simulink model "OpenLoop"  (Simulink 10.2)
settings: Solver=ode4  StartTime=0.0  StopTime=TMax  FixedStep=DT  MaxStep=DT  RelTol=1e-3  EnableMultiTasking=on
undefined symbols (not defined in the file or in its folder): OutList, sigbuilder_block, strmatch
settings Model: LogicAnalyzerSignalOrdering=622969c7-4a95-484c-aa48-d70039800655,567f855e-93bb-40e6-82fe-fffaa7f8c6d2,f9a8c3cb-64e9-4f89-868b-cd3825c112bf,cfa72df4-fa35-4a41-bc9f-f1a82cc1069a,cd711ec8-28aa-4c52-819f-5cc7fce55bd0  Creator=bjonkman  LastModifiedBy=oster
settings DataIOCC: LimitDataPoints=on  SaveOutput=off  SaveTime=off  SignalLoggingName=sigsOut
settings OptimizationCC: ExpressionDepthLimit=2147483647
settings DebuggingCC: SaveWithParameterizedLinksMsg=none  SignalResolutionControl=TryResolveAllWithWarning  MultiTaskDSMMsg=warning  MultiTaskCondExecSysMsg=none  StateNameClashWarn=warning
settings HardwareCC: TargetUnknown=on

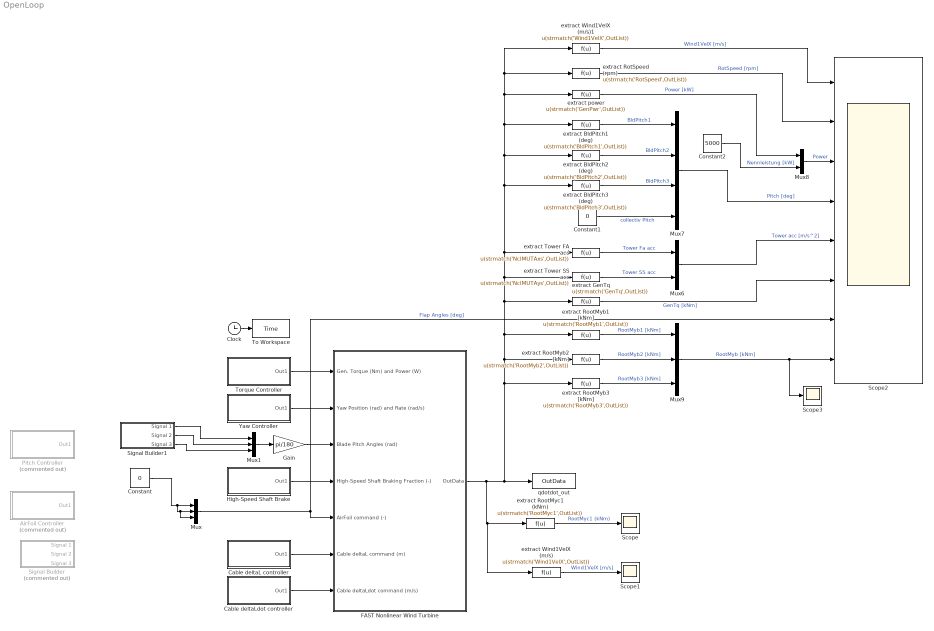
== system OpenLoop ==
  AirFoil Controller : Subsystem  Commented=on
  Cable deltaL controller : Subsystem
  Cable deltaLdot controller : Subsystem
  Clock : Clock
  Constant : Constant  Value=0
  Constant1 : Constant  Value=0
  Constant2 : Constant  Value=5000
  FAST Nonlinear Wind Turbine : Subsystem  mask(FAST Nonlinear Wind Turbine){}
      mask help: This block contains the FAST S-Function.
      mask init:
      | clear FAST_SFunc
  Gain : Gain  Gain=pi/180
  High-Speed Shaft Brake : Subsystem
  Mux : Mux  Inputs=3
  Mux1 : Mux  Inputs=3
  Mux6 : Mux  Inputs=2
  Mux7 : Mux
  Mux8 : Mux  Inputs=2
  Mux9 : Mux  Inputs=3
  Pitch Controller : Subsystem  Commented=on
  Scope : Scope
  Scope1 : Scope
  Scope2 : Scope  NumInputPorts=8
  Scope3 : Scope
  Signal Builder : Subsystem  Tag=STV Subsys  Commented=on  LoadFcn=sigbuilder_block('load');  StartFcn=sigbuilder_block('start');  StopFcn=sigbuilder_block('stop');  ClipboardFcn=sigbuilder_block('clipboard');  mask(Sigbuilder block){tuvar=[0:10]}
      mask help: Simulink:masks:SigbuilderBlock_MD
      mask init:
      | if ~strcmp(get_param(bdroot(gcbh),'SimulationStatus'),'stopped') tuvar = sigbuilder_block('maskInit'); end
      settings: CopyFcn=sigbuilder_block('copy');  DeleteFcn=sigbuilder_block('delete');  ModelCloseFcn=sigbuilder_block('modelClose');  PreSaveFcn=sigbuilder_block('preSave');  PauseFcn=sigbuilder_block('pause');  ContinueFcn=sigbuilder_block('continue');  NameChangeFcn=sigbuilder_block('namechange');  OpenFcn=sigbuilder_block('open',[1778.25 246.75 675 420.75 ]);  CloseFcn=sigbuilder_block('close');
      mask Display: plot(0, 0, 100, 100,[2, 2, 32, 32, 2], [68, 8, 8, 68, 68],[32, 2], [38, 38], [32, 19, 2],[53, 60, 44], [32, 17, 17, 2],[16, 16, 31, 31]);txt = getActiveGroup(gcbh);text(2, 100, txt,'verticalAlignment', 'top');
  Signal Builder1 : Subsystem  Tag=STV Subsys  LoadFcn=sigbuilder_block('load');  StartFcn=sigbuilder_block('start');  StopFcn=sigbuilder_block('stop');  ClipboardFcn=sigbuilder_block('clipboard');  mask(Sigbuilder block){tuvar=[0:10]}
      mask help: Simulink:masks:SigbuilderBlock_MD
      mask init:
      | if ~strcmp(get_param(bdroot(gcbh),'SimulationStatus'),'stopped') tuvar = sigbuilder_block('maskInit'); end
      settings: CopyFcn=sigbuilder_block('copy');  DeleteFcn=sigbuilder_block('delete');  ModelCloseFcn=sigbuilder_block('modelClose');  PreSaveFcn=sigbuilder_block('preSave');  PauseFcn=sigbuilder_block('pause');  ContinueFcn=sigbuilder_block('continue');  NameChangeFcn=sigbuilder_block('namechange');  OpenFcn=sigbuilder_block('open',[1778.25 246.75 675 420.75 ]);  CloseFcn=sigbuilder_block('close');
      mask Display: plot(0, 0, 100, 100,[2, 2, 32, 32, 2], [68, 8, 8, 68, 68],[32, 2], [38, 38], [32, 19, 2],[53, 60, 44], [32, 17, 17, 2],[16, 16, 31, 31]);txt = getActiveGroup(gcbh);text(2, 100, txt,'verticalAlignment', 'top');
  To Workspace : ToWorkspace  VariableName=Time  SampleTime=-1
  Torque Controller : Subsystem
  Yaw Controller : Subsystem
  extract BldPitch1 (deg) : Fcn  Expr=u(strmatch('BldPitch1',OutList))
  extract BldPitch2 (deg) : Fcn  Expr=u(strmatch('BldPitch2',OutList))
  extract BldPitch3 (deg) : Fcn  Expr=u(strmatch('BldPitch3',OutList))
  extract GenTq : Fcn  Expr=u(strmatch('GenTq',OutList))
  extract RootMyb1 [kNm] : Fcn  Expr=u(strmatch('RootMyb1',OutList))
  extract RootMyb2 [kNm] : Fcn  Expr=u(strmatch('RootMyb2',OutList))
  extract RootMyb3 [kNm] : Fcn  Expr=u(strmatch('RootMyb3',OutList))
  extract RootMyc1 (kNm) : Fcn  Expr=u(strmatch('RootMyc1',OutList))
  extract RotSpeed (rpm) : Fcn  Expr=u(strmatch('RotSpeed',OutList))
  extract Tower FA acc : Fcn  Expr=u(strmatch('NcIMUTAxs',OutList))
  extract Tower SS acc : Fcn  Expr=u(strmatch('NcIMUTAys',OutList))
  extract Wind1VelX (m/s) : Fcn  Expr=u(strmatch('Wind1VelX',OutList))
  extract Wind1VelX (m/s)1 : Fcn  Expr=u(strmatch('Wind1VelX',OutList))
  extract power : Fcn  Expr=u(strmatch('GenPwr',OutList))
  qdotdot_out : ToWorkspace  VariableName=OutData  SampleTime=-1
  wires:
  Clock/1 -> To Workspace/1
  Torque Controller/1(Out1) -> FAST Nonlinear Wind Turbine/1(Gen. Torque (Nm) and Power (W))
  Yaw Controller/1(Out1) -> FAST Nonlinear Wind Turbine/2(Yaw Position (rad) and Rate (rad/s))
  Mux1/1 -> Gain/1
  High-Speed Shaft Brake/1(Out1) -> FAST Nonlinear Wind Turbine/4(High-Speed Shaft Braking Fraction (-))
  Cable deltaL controller/1(Out1) -> FAST Nonlinear Wind Turbine/6(Cable deltaL command (m))
  Cable deltaLdot controller/1(Out1) -> FAST Nonlinear Wind Turbine/7(Cable deltaLdot command (m/s))
  extract RootMyc1 (kNm)/1 -> Scope/1  "RootMyc1 (kNm)"
  extract Wind1VelX (m/s)/1 -> Scope1/1  "Wind1VelX [m/s]"
  extract Tower FA acc/1 -> Mux6/1  "Tower Fa acc"
  extract BldPitch2 (deg)/1 -> Mux7/2  "BldPitch2"
  extract Wind1VelX (m/s)1/1 -> Scope2/1  "Wind1VelX [m/s]"
  extract GenTq/1 -> Scope2/6  "GenTq [kNm]"
  extract RootMyb1 [kNm]/1 -> Mux9/1  "RootMyb1 [kNm]"
  Mux6/1 -> Scope2/5  "Tower acc [m/s^2]"
  extract RootMyb3 [kNm]/1 -> Mux9/3  "RootMyb3 [kNm]"
  extract BldPitch1 (deg)/1 -> Mux7/1  "BldPitch1"
  extract RotSpeed (rpm)/1 -> Scope2/2  "RotSpeed [rpm]"
  extract BldPitch3 (deg)/1 -> Mux7/3  "BldPitch3"
  extract Tower SS acc/1 -> Mux6/2  "Tower SS acc"
  FAST Nonlinear Wind Turbine/1(OutData) -> extract Wind1VelX (m/s)/1, extract RootMyc1 (kNm)/1, extract RootMyb3 [kNm]/1, extract RootMyb1 [kNm]/1, extract GenTq/1, extract Tower SS acc/1, extract Tower FA acc/1, extract RotSpeed (rpm)/1, extract Wind1VelX (m/s)1/1, extract power/1, extract BldPitch1 (deg)/1, extract BldPitch2 (deg)/1, extract BldPitch3 (deg)/1, extract RootMyb2 [kNm]/1, qdotdot_out/1
  Constant1/1 -> Mux7/4  "collectiv Pitch"
  Constant2/1 -> Mux8/2  "Nennleistung [kW]"
  Mux/1 -> FAST Nonlinear Wind Turbine/5(AirFoil command (-)), Scope2/7  "Flap Angles [deg]"
  extract RootMyb2 [kNm]/1 -> Mux9/2  "RootMyb2 [kNm]"
  Mux9/1 -> Scope3/1, Scope2/8  "RootMyb [kNm]"
  extract power/1 -> Mux8/1  "Power [kW]"
  Mux8/1 -> Scope2/3  "Power"
  Mux7/1 -> Scope2/4  "Pitch [deg]"
  Signal Builder1/3(Signal 3) -> Mux1/3
  Signal Builder1/2(Signal 2) -> Mux1/2
  Signal Builder1/1(Signal 1) -> Mux1/1
  Constant/1 -> Mux/3, Mux/2, Mux/1
  Gain/1 -> FAST Nonlinear Wind Turbine/3(Blade Pitch Angles (rad))

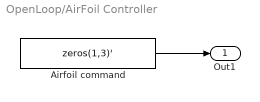
== system OpenLoop/AirFoil Controller ==
  Airfoil command : Constant  Value=zeros(1,3)'
  Out1 : Outport
  wires:
  Airfoil command/1 -> Out1/1

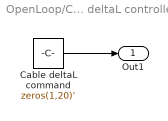
== system OpenLoop/Cable deltaL controller ==
  Cable deltaL command : Constant  Value=zeros(1,20)'
  Out1 : Outport
  wires:
  Cable deltaL command/1 -> Out1/1

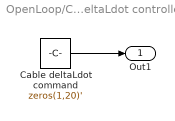
== system OpenLoop/Cable deltaLdot controller ==
  Cable deltaLdot command : Constant  Value=zeros(1,20)'
  Out1 : Outport
  wires:
  Cable deltaLdot command/1 -> Out1/1

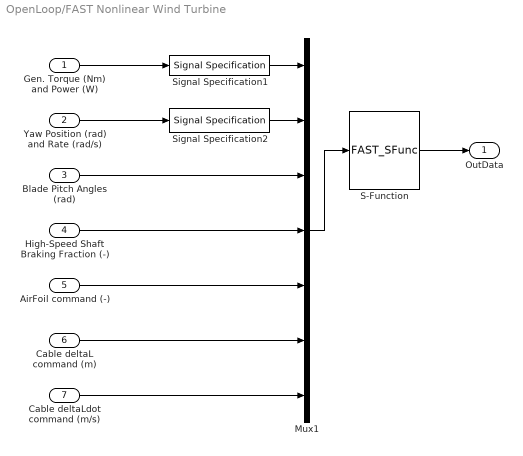
== system OpenLoop/FAST Nonlinear Wind Turbine ==
  Gen. Torque (Nm) and Power (W) : Inport
  Yaw Position (rad) and Rate (rad/s) : Inport  Port=2
  Blade Pitch Angles (rad) : Inport  Port=3
  High-Speed Shaft Braking Fraction (-) : Inport  Port=4
  AirFoil command (-) : Inport  Port=5
  Cable deltaL command (m) : Inport  Port=6
  Cable deltaLdot command (m/s) : Inport  Port=7
  Mux1 : Mux  Inputs=7
  S-Function : S-Function  FunctionName=FAST_SFunc  Parameters=FAST_InputFileName, TMax, 0  SFunctionDeploymentMode=off  EnableBusSupport=off
  Signal Specification1 : SignalSpecification  OutDataTypeStr=double  Dimensions=2
  Signal Specification2 : SignalSpecification  OutDataTypeStr=double  Dimensions=2
  OutData : Outport
  wires:
  Gen. Torque (Nm) and Power (W)/1 -> Signal Specification1/1
  S-Function/1 -> OutData/1
  Mux1/1 -> S-Function/1
  Blade Pitch Angles (rad)/1 -> Mux1/3
  Yaw Position (rad) and Rate (rad/s)/1 -> Signal Specification2/1
  Signal Specification1/1 -> Mux1/1
  Signal Specification2/1 -> Mux1/2
  High-Speed Shaft Braking Fraction (-)/1 -> Mux1/4
  AirFoil command (-)/1 -> Mux1/5
  Cable deltaL command (m)/1 -> Mux1/6
  Cable deltaLdot command (m/s)/1 -> Mux1/7

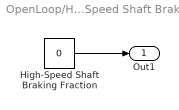
== system OpenLoop/High-Speed Shaft Brake ==
  High-Speed Shaft Braking Fraction : Constant  Value=0
  Out1 : Outport
  wires:
  High-Speed Shaft Braking Fraction/1 -> Out1/1

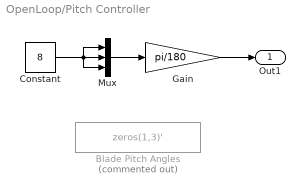
== system OpenLoop/Pitch Controller ==
  Blade Pitch Angles : Constant  Commented=on  Value=zeros(1,3)'
  Constant : Constant  Value=8
  Gain : Gain  Gain=pi/180
  Mux : Mux  Inputs=3
  Out1 : Outport
  wires:
  Constant/1 -> Mux/2, Mux/3, Mux/1
  Mux/1 -> Gain/1
  Gain/1 -> Out1/1

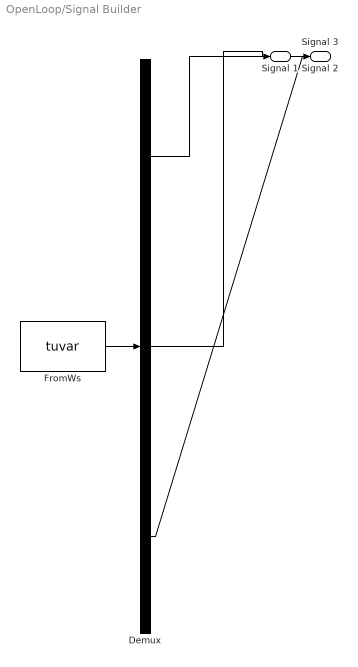
== system OpenLoop/Signal Builder ==
  Demux : Demux  Tag=STV Demux  Outputs=3
      settings: DisplayOption=none
  FromWs : FromWorkspace  Tag=STV FromWs  VariableName=tuvar  SigBuilderData=DataTag0  VnvData=DataTag1
      SigBuilderData=|
      | common.afterFinalStr = 'Extrapolate'
      | common.sampleTime = 0
      | dataSet.timeRange = [0 60]
      | dataSet.name = 'Group 1'
      | sbobj.Groups.Name = 'Group 1'
      | sbobj.Groups.Signals(1).Name = 'Signal 1'
      | sbobj.Groups.Signals(1).XData = [0 15.7 15.7 23.3 23.3 60]
      | sbobj.Groups.Signals(1).YData = [0 0 10 10 0 0]
      | sbobj.Groups.Signals(2).Name = 'Signal 2'
      | sbobj.Groups.Signals(2).XData = [0 29.4 29.4 36 36 60]
      | sbobj.Groups.Signals(2).YData = [0 0 1 1 0 0]
      | sbobj.Groups.Signals(3).Name = 'Signal 3'
      | sbobj.Groups.Signals(3).XData = [0 43.4 43.4 50.8 50.8 60]
      | sbobj.Groups.Signals(3).YData = [0 0 -5.1 -5.1 0 0]
      | sbobj.Groups.TimeRange = [0 60]
  Signal 1 : Outport  Tag=STV Outport
  Signal 2 : Outport  Tag=STV Outport  Port=2
  Signal 3 : Outport  Tag=STV Outport  Port=3
  wires:
  Demux/1 -> Signal 1/1
  FromWs/1 -> Demux/1
  Demux/2 -> Signal 2/1
  Demux/3 -> Signal 3/1

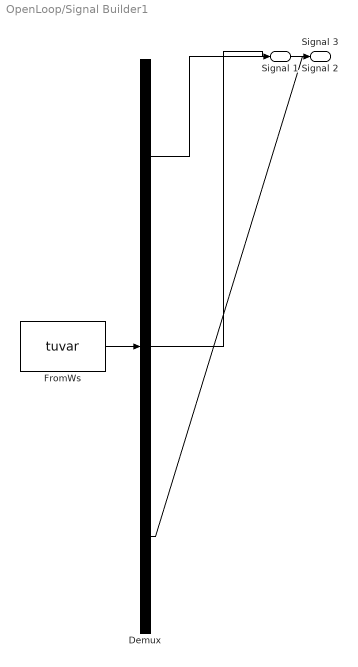
== system OpenLoop/Signal Builder1 ==
  Demux : Demux  Tag=STV Demux  Outputs=3
      settings: DisplayOption=none
  FromWs : FromWorkspace  Tag=STV FromWs  VariableName=tuvar  SigBuilderData=DataTag2  VnvData=DataTag3
      SigBuilderData=|
      | common.afterFinalStr = 'Extrapolate'
      | common.sampleTime = 0
      | dataSet.timeRange = [0 60]
      | dataSet.name = 'Group 1'
      | sbobj.Groups.Name = 'Group 1'
      | sbobj.Groups.Signals(1).Name = 'Signal 1'
      | sbobj.Groups.Signals(1).XData = [0 15.7 15.7 23.3 23.3 60]
      | sbobj.Groups.Signals(1).YData = [0 0 10 10 0 0]
      | sbobj.Groups.Signals(2).Name = 'Signal 2'
      | sbobj.Groups.Signals(2).XData = [0 29.4 29.4 36 36 60]
      | sbobj.Groups.Signals(2).YData = [0 0 1 1 0 0]
      | sbobj.Groups.Signals(3).Name = 'Signal 3'
      | sbobj.Groups.Signals(3).XData = [0 43.4 43.4 50.8 50.8 60]
      | sbobj.Groups.Signals(3).YData = [0 0 -5.1 -5.1 0 0]
      | sbobj.Groups.TimeRange = [0 60]
  Signal 1 : Outport  Tag=STV Outport
  Signal 2 : Outport  Tag=STV Outport  Port=2
  Signal 3 : Outport  Tag=STV Outport  Port=3
  wires:
  Demux/3 -> Signal 3/1
  Demux/2 -> Signal 2/1
  FromWs/1 -> Demux/1
  Demux/1 -> Signal 1/1

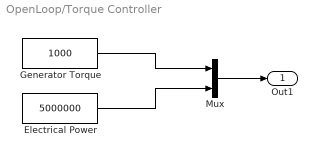
== system OpenLoop/Torque Controller ==
  Electrical Power : Constant  Value=5000000
  Generator Torque : Constant  Value=1000
  Mux : Mux  Inputs=2
  Out1 : Outport
  wires:
  Mux/1 -> Out1/1
  Generator Torque/1 -> Mux/1
  Electrical Power/1 -> Mux/2

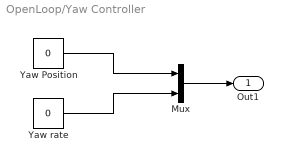
== system OpenLoop/Yaw Controller ==
  Mux : Mux  Inputs=2
  Yaw Position : Constant  Value=0
  Yaw rate : Constant  Value=0
  Out1 : Outport
  wires:
  Mux/1 -> Out1/1
  Yaw Position/1 -> Mux/1
  Yaw rate/1 -> Mux/2
